simulink model "ssc_bridge_rectifier_rt_2_sc_display"  (R2021b)
settings: Solver=ode3  StartTime=0.0  StopTime=0.05  FixedStep=0.0001  MaxStep=0.001  RelTol=1e-3
PostLoadFcn:
  | Ts=100e-6;
InitFcn:
  | Ts=100e-6;
libraries: opal_lib x3
Description:
  | Full-Wave Bridge Rectifier
  | 
  | This is a model of a power supply that converts 120 volts AC to 12  volts DC. The
  | transformer has a turns ratio of 14, stepping the supply down to 8.6 volts rms, i.e.
  | 8.6*sqrt(2) = 12 volts pk-pk. The full-wave bridge rectifier plus capacitor combination
  | then converts this to DC. The resistor represents a typical load.
  | 
  | The model can be used to size the capacitor required for a specified load.  For a
  | given size of capacitor, as the load resistance is increased, the ripple on the DC
  | voltage increases. The model can also be used to drive an application circuit in
  | order to assess the effect of the ripple.
  | 
  | 
  | Copyright 2008 The MathWorks(TM), Inc.
settings Model: Creator=rhyde  LastModifiedBy=fghow
settings SolverCC: AlgebraicLoopSolver=TrustRegion
settings DataIOCC: LimitDataPoints=on  SaveFormat=Array  SignalLoggingSaveFormat=ModelDataLogs  SaveOutput=off  SignalLogging=off  SaveTime=off  ReturnWorkspaceOutputs=off
settings OptimizationCC: BlockReduction=off  OptimizeBlockIOStorage=off  BufferReuse=off  ExpressionFolding=off  ExpressionDepthLimit=2147483647  LocalBlockOutputs=off  InitFltsAndDblsToZero=on  LifeSpan=inf
settings DebuggingCC: SaveWithParameterizedLinksMsg=none  UnderspecifiedInitializationDetection=Classic  MergeDetectMultiDrivingBlocksExec=none  SignalResolutionControl=TryResolveAllWithWarning  SolverPrmCheckMsg=warning  FcnCallInpInsideContextMsg=warning  StateNameClashWarn=warning  SFUnexpectedBacktrackingDiag=warning  SFNoUnconditionalDefaultTransitionDiag=warning  SFExecutionAtInitializationDiag=none  SFMachineParentedDataDiag=warning  ArithmeticOperatorsInVariantConditions=warning
settings HardwareCC: ProdBitPerPointer=32  ProdBitPerSizeT=32  ProdBitPerPtrDiffT=32  ProdLargestAtomicFloat=None  ProdIntDivRoundTo=Undefined  ProdEndianess=Unspecified  ProdWordSize=32  ProdHWDeviceType=32-bit Generic
settings ModelReferenceCC: PropagateSignalLabelsOutOfModel=off
settings SFSimCC: SimUseLocalCustomCode=off  CustomCodeUndefinedFunction=UseInterfaceOnly
settings RTWCC: GenCodeOnly=on  RTWUseLocalCustomCode=off
settings CodeAppCC: StateflowObjectComments=on
settings GRTTargetCC: TargetFcnLib=ansi_tfl_tmw.mat  TargetLangStandard=C89/C90 (ANSI)  CombineOutputUpdateFcns=off  GRTInterface=on
settings ConfigComp: CovMetricSettings=dw  CovSaveCumulativeToWorkspaceVar=on  CovSaveSingleToWorkspaceVar=on  CovExternalEMLEnable=off
settings SimscapeCC: SimscapeNormalizeSystem=off

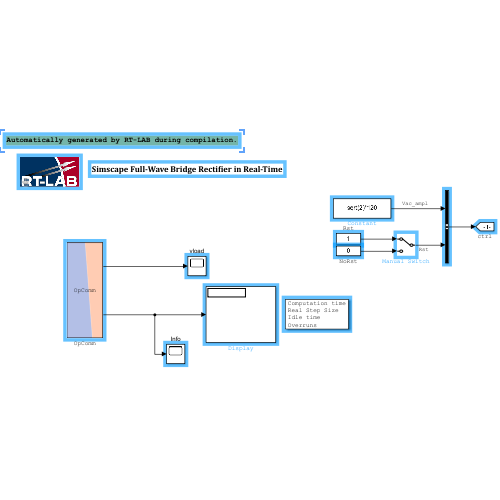
[thumbnail: Simulink's stored preview of the top-level diagram]
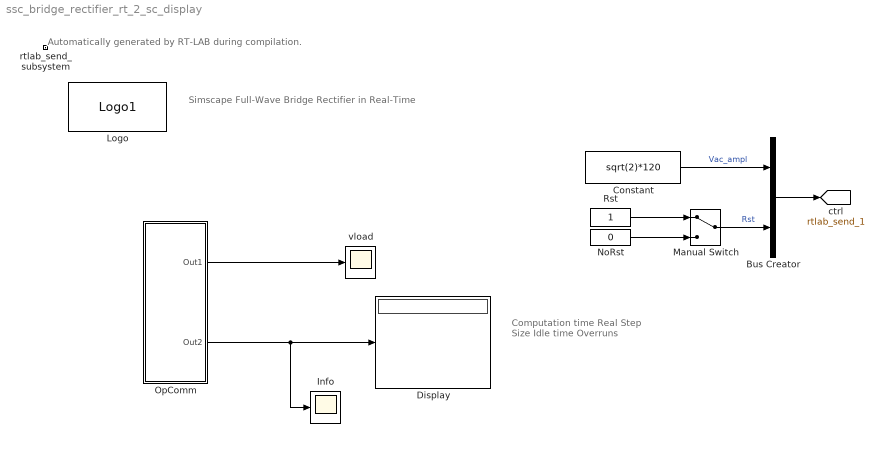
== system ssc_bridge_rectifier_rt_2_sc_display ==
  note: Automatically generated by RT-LAB during compilation.
  note: Simscape Full-Wave Bridge Rectifier in Real-Time
  note: Computation time
      | Real Step Size
      | Idle time
      | Overruns
  Bus Creator : BusCreator  Inputs=2
  Constant : Constant  Value=sqrt(2)*120
  Display : Display
  Info : Scope
  Logo : opal_lib/Logo1  vide=[]
  Manual Switch : ManualSwitch
  NoRst : Constant  Value=0
  OpComm : Subsystem
      mask init:
      | opmaskdisplay('maskdisplay_block',gcb,'disp(''OpComm'')');
      mask Display:
      | patch([0 0.5 0.7 0],[1 1 0 0],[0.7 0.75 0.9]);
      | patch([1 0.53 0.73 1],[1 1 0 0],[1 0.8 0.7]);
      | plot([0 0 1 1 0],[0 1 1 0 0]);
      | disp('OpComm')
  Rst : Constant
  rtlab_send_subsystem : Subsystem  Priority=-100
      mask Display: text(0,0,'');
  vload : Scope
  tag scope: rtlab_send_1=global
  wires:
  Manual Switch/1 -> Bus Creator/2  "Rst"
  Constant/1 -> Bus Creator/1  "Vac_ampl"
  Bus Creator/1 -> [rtlab_send_1]
  NoRst/1 -> Manual Switch/2
  Rst/1 -> Manual Switch/1
  OpComm/2(Out2) -> Info/1, Display/1
  OpComm/1(Out1) -> vload/1

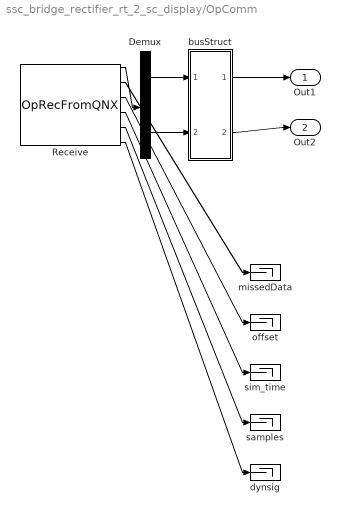
== system ssc_bridge_rectifier_rt_2_sc_display/OpComm ==
  Demux : Demux  Outputs="[1  4]"
  Receive : opal_lib/Communication/OpRecFromQNX  Node_num=1  Acqu_Group=1  Data_Width=5  Synchronization=on  Interpolation=on  Threshold=1.0  modelname=ssc_bridge_rectifier_rt  sampletime=0.0001
  busStruct : Subsystem
  dynsig : Terminator
  missedData : Terminator
  offset : Terminator
  samples : Terminator
  sim_time : Terminator
  Out1 : Outport
  Out2 : Outport  Port=2
  wires:
  Demux/2 -> busStruct/2(In2)
  Demux/1 -> busStruct/1(In1)
  busStruct/2(Out2) -> Out2/1
  busStruct/1(Out1) -> Out1/1
  Receive/1 -> Demux/1
  Receive/6 -> dynsig/1
  Receive/5 -> samples/1
  Receive/4 -> sim_time/1
  Receive/3 -> offset/1
  Receive/2 -> missedData/1

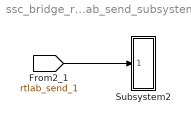
== system ssc_bridge_rectifier_rt_2_sc_display/rtlab_send_subsystem ==
  Subsystem2 : Subsystem
  wires:
  [rtlab_send_1] -> Subsystem2/1(In1)

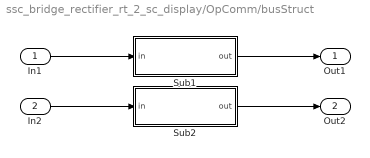
== system ssc_bridge_rectifier_rt_2_sc_display/OpComm/busStruct ==
  In1 : Inport
  In2 : Inport  Port=2
  Sub1 : Subsystem
  Sub2 : Subsystem
  Out1 : Outport
  Out2 : Outport  Port=2
  wires:
  Sub2/1(out) -> Out2/1
  In2/1 -> Sub2/1(in)
  Sub1/1(out) -> Out1/1
  In1/1 -> Sub1/1(in)

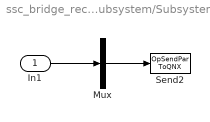
== system ssc_bridge_rectifier_rt_2_sc_display/rtlab_send_subsystem/Subsystem2 ==
  In1 : Inport  PortDimensions=2
  Mux : Mux  Inputs=1
  Send2 : opal_lib/Communication/OpSendPar ToQNX  Node_num=1  modelname=ssc_bridge_rectifier_rt
  wires:
  Mux/1 -> Send2/1
  In1/1 -> Mux/1

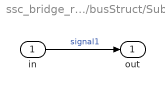
== system ssc_bridge_rectifier_rt_2_sc_display/OpComm/busStruct/Sub1 ==
  in : Inport
  out : Outport
  wires:
  in/1 -> out/1  "signal1"

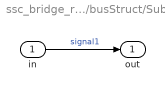
== system ssc_bridge_rectifier_rt_2_sc_display/OpComm/busStruct/Sub2 ==
  in : Inport
  out : Outport
  wires:
  in/1 -> out/1  "signal1"
